simulink model "Final_Model"  (R2020a)
settings: Solver=VariableStepAuto  StartTime=0.0  StopTime=15  RelTol=1e-3
model workspace (MAT data in the model file):
  breaker_state = Simulink.Parameter
  breaker_state.Value = 0
  breaker_state.DataType = 'auto'
  breaker_state.Dimensions = [1 1]
  cap_state = Simulink.Parameter
  cap_state.Value = 1
  cap_state.DataType = 'double'
  cap_state.Dimensions = [1 1]
undefined symbols (not defined in the file or in its folder): state
libraries: ee_lib x78, nesl_utility x49, fl_lib x10, simulink x2
(part 1 of 2)
settings Model: OrderedModelArguments=off  Creator=mrinm  LastModifiedBy=HP

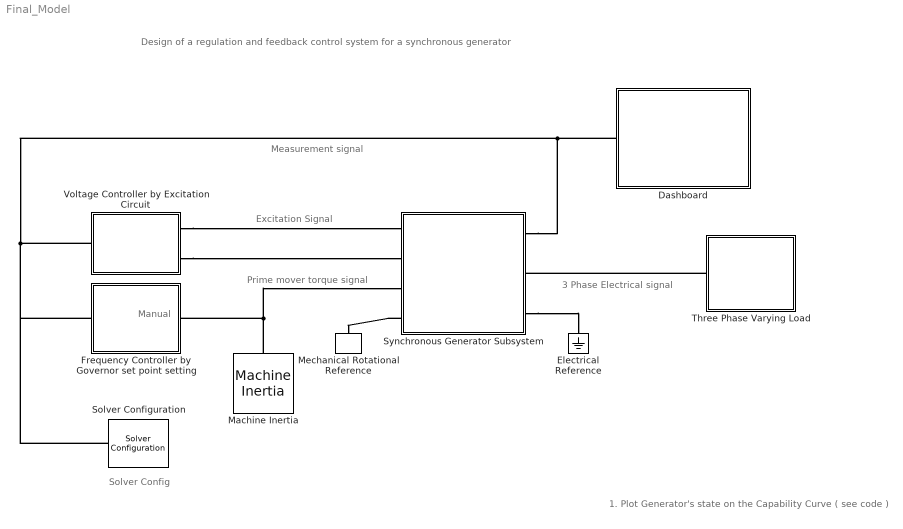
== system Final_Model ==
  note: Design of a regulation and feedback control system
      | for a synchronous generator
  note: 3 Phase Electrical signal
  note: 1. Plot Generator's state on the Capability Curve ( see code )
  note: Manual
  note: Measurement signal
  note: Excitation Signal
  note: Prime mover torque signal
  note: Solver Config
  Dashboard : Subsystem
      mask Display: image("images/dashboard.png")
  Electrical Reference : fl_lib/Electrical/Electrical Elements/Electrical Reference
      settings: SourceProductBaseCode=MT,SS
  Frequency Controller by Governor set point setting : Subsystem  mask(Governor and Prime Mover){pu_speed_reference=1, droop_percentage=10, T_G=0.2, T_CH=0.3, base_torque=2.65258e+06, pu_torque0=0.451059}
      mask prompts: pu_speed_reference "Speed reference, (pu)"; droop_percentage "Percentage droop, (%)"; T_G "Time constant of governor, (s)"; T_CH "Time constant of turbine T_CH, (s)"; base_torque "Base torque, (N*m)"; pu_torque0 "Initial torque, (pu)"
      mask help:
      | Implements a synchronous machine governor and prime mover.
      |
      | The governor response is modelled by a 1st order transfer function with time constant T_G. Likewise the prime mover also is a modelled by 1st order transfer function with time constant T_CH.
      |
      | The input to the block is a per-unit synchronous machine measurement vector.
      |
      | R and C are mechanical rotational ports.
      |
      | The stabilization of the rotor speed is implemented by a discrete PID controller which takes a reference speed and the pu_rotor_speed as input to calculate optimum governor set point value. The PID controller was tuned with Simulink auto tuner beforehand.
  Machine Inertia : ee_lib/Electromechanical/Mechanical/Machine Inertia  SRated=555e6 V*A  FRated=60 Hz  nPolePairs=1  inertia_option=2  J=27548 kg*m^2  H=3.525 s*W/V/A  damper_option=2  D=39.0509 N*m/(rad/s)  pu_D=0.01  initialization_option=2  fMechanical0=60 Hz  fElectrical0=60 Hz
      settings: SourceProductBaseCode=PS  InternalSimscapePortConfiguration="{\"Bottom\":[],\"Left\":[{\"id\":\"R\",\"label\":\"R\",\"type\":\"foundation.mechanical.rotational.rotational\"}],\"Right\":[],\"Top\":[]}"
  Mechanical Rotational Reference : fl_lib/Mechanical/Rotational Elements/Mechanical Rotational Reference
      settings: SourceProductBaseCode=MT,SS
  Solver Configuration : nesl_utility/Solver Configuration  PhysicalDomain=network_engine_domain  SubClassName=solver  LeftPortType=input  RightPortType=generic  Tones=[]  Harmonics=[]  SimulateNoise=off  Profile=off  UseLocalSampling=off  EnableSwitchedLinearOptims=on  FrequencyDomain=off  UseCCode=off  RelTol=0.001  AbsTol=1e-06  MinStep=1e-09  ToWorkspace=off  RevertToSquareIcSolve=off  NumHomotopyIterations=100  PhasorMode=off  PhasorModeNumHarmonics=1  DoDC=off  ResidualTolerance=1e-09  UseLocalSolver=on  LocalSolverChoice=NE_BACKWARD_EULER_ADVANCER  LocalSolverSampleTime=1e-3  DoFixedCost=on  MaxNonlinIter=3  MaxModeIter=2  LinearAlgebra=auto  EquationFormulation=NE_TIME_EF  DelaysMemoryBudget=1024  AutomaticFiltering=on  FilteringTimeConstant=0.001  PartitionStorageMethod=AS_NEEDED  PartitionMemoryBudget=1024  PartitionMethod=FAST
      settings: SourceProductBaseCode=MT,SS
  Synchronous Generator Subsystem : Subsystem
      mask Display: image("images/generator.jpg")
  Three Phase Varying Load : Subsystem  mask{load_type=3.Increasing Lagging, vrated=24e3, frated=60, varated=555e6}
      mask prompts: load_type "Select Load"; vrated "Rated Voltage"; frated "Rated Frequency"; varated "VA ratings"
      mask help:
      | The 3 phase load is a combination of multiple loads seen in a typical power system. A practical load is a function of time. The loads are modeled in this component.The load types are:
      | 1. Increasing Unity: A load with unity powerfactor and increasing magnitude(VA)
      | 2. Increasing Leading: A fully leading load with increasing magnitude(VA)
      | 3. Increasing Lagging: A fully lagging load with increasing magnitude(VA)
      | 4. Leading to Lagging: A load with increasing powerfactor
      | 5. Lagging to Leading: A load with decreasing powerfactor
      | 6. Varying Load: A load which VA is changing over time.
      | 7. Overload: A load bigger than the rated load.
      |
      | (Loads are not continuously time varying. Their variation is discrete.)
      mask init:
      | global state
      mask TypeOptions load_type: 1.Increasing Unity | 2.Increasing Leading | 3.Increasing Lagging | 4.Leading to Lagging | 5.Lagging to Leading | 6.Varying load | 7.Overload
      mask Callback load_type:
      | maskStr = get_param(gcb,'load_type');
      | global state
      | state=[1 1 1 1 1 1 1 1 1 1];
      | % The pop-up menu is the first mask parameter.
      | %   Check the value selected in the pop-up
      | if strcmp(maskStr(1),'1'),
      |     state(1) = 0;
      | elseif strcmp(maskStr(1),'2'),
      |     state(2) = 0;
      | elseif strcmp(maskStr(1),'3'),
      |     state(3) = 0;
      | elseif strcmp(maskStr(1),'4'),
      |     state(4) = 0;
      | elseif strcmp(maskStr(1),'5'),
      |     state(5) = 0;
      | elseif strcmp(maskStr(1),'6'),
      |     state(6) = 0;
      | elseif strcmp(maskStr(1),'7'),
      |     state(7) = 0;
      | elseif strcmp(maskStr(1),'8'),
      |     state(8) = 0;
      | elseif strcmp(maskStr(1),'9'),
      |     state(9) = 0;
      | else
      |     state(10) = 0;
      | 
      |     % Turn off the visibility of the Value field
      |     %   when User-defined is not selected.
      | 
      | 
      | 
      |     % Set the character vector in the Values field equal to the
      |     % character vector selected in the Gain pop-up menu.
      | 
      |     %maskStr{2}=maskStr{1};
      |     %set_param(gcb,'editvalue',maskStr);
      | end
      | disp(state);
      mask Display: image("images/electric_load.jpg")
  Voltage Controller by Excitation Circuit : Subsystem  mask{Vref=1, Tr=0, Ka=50, Ta=0.070, Kf=0.05, Tf=1.040, Te=0.703}
      mask prompts: Vref "Reference Voltage Vref(pu)"; Tr "Tranducer Time Constant Tr(s)"; Ka "Regulator Gain Ka(10-400)"; Ta "AVR Time Constant Ta(s)"; Kf "Feedback Gain Kf(0.03-0.1)"; Tf "Feedback Time Constant Tf(s)"; Te "Exciter Time Constant Te(s)"
      mask DialogControl DescGroupVar Prompt: Voltage Controller(mask)
      mask DialogControl DescTextVar Prompt: The input to the block is a per-unit synchronous machine measurement vector. fd+ & fd- are the positive & negative terminal field voltage
  connections:
  Machine Inertia/LConn1 -- Synchronous Generator Subsystem/LConn3 -- Frequency Controller by Governor set point setting/RConn1
  Synchronous Generator Subsystem/RConn1 -- Frequency Controller by Governor set point setting/LConn1 -- Solver Configuration/RConn1 -- Voltage Controller by Excitation Circuit/LConn1 -- Dashboard/LConn1
  Voltage Controller by Excitation Circuit/RConn1 -- Synchronous Generator Subsystem/LConn1
  Voltage Controller by Excitation Circuit/RConn2 -- Synchronous Generator Subsystem/LConn2
  Synchronous Generator Subsystem/LConn4 -- Mechanical Rotational Reference/LConn1
  Synchronous Generator Subsystem/RConn3 -- Electrical Reference/LConn1
  Three Phase Varying Load/LConn1 -- Synchronous Generator Subsystem/RConn2

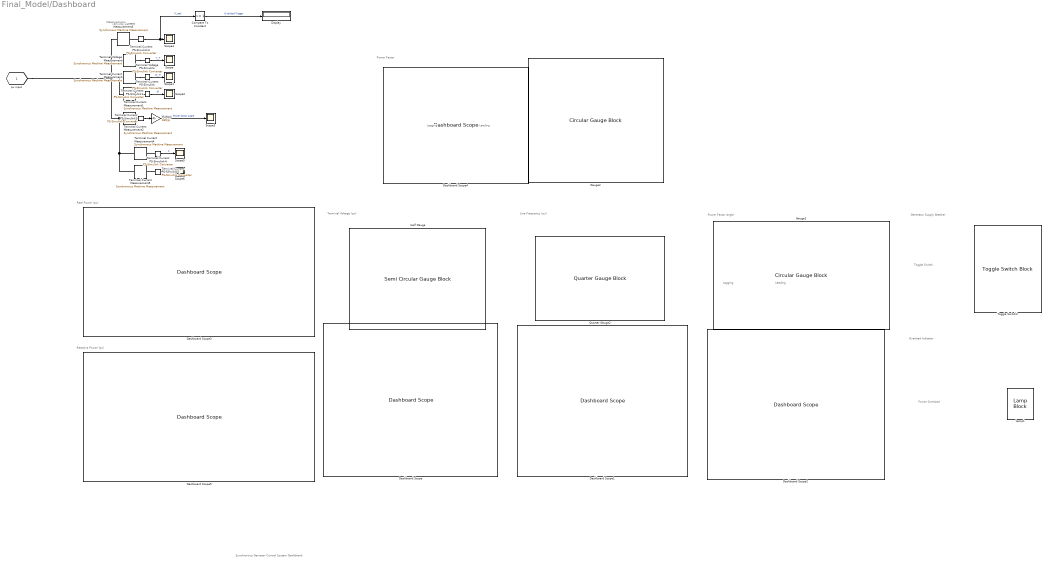
== system Final_Model/Dashboard ==
  note: Power Overload
  note: Lagging
  note: Leading
  note: Terminal Voltage (pu)
  note: Line Frequency (pu)
  note: Synchronous Genrator Control System Dashboard
  note: Power Factor Angle
  note: Leading
  note: Lagging
  note: Power Factor
  note: Real Power (pu)
  note: Overload Indicator
  note: Generator Supply Breaker
  note: Measurement
  note: Toggle Switch
  note: Reactive Power (pu)
  Compare To Constant : simulink/Logic and Bit Operations/Compare To Constant  relop=>=  const=1  OutDataTypeStr=uint8
  Dashboard Scope : DashboardScope  Ymin=0  Ymax=2  LegendPosition=Hide  ScaleAtStop=off
  Dashboard Scope1 : DashboardScope  Ymin=.9  Ymax=1.1  LegendPosition=Hide  ScaleAtStop=off
  Dashboard Scope2 : DashboardScope  Ymin=-90  Ymax=90  LegendPosition=Hide  ScaleAtStop=off
  Dashboard Scope3 : DashboardScope  Ymin=0  Ymax=2  ScaleAtStop=off
  Dashboard Scope4 : DashboardScope  Ymin=0  Ymax=1.2  LegendPosition=Hide  ScaleAtStop=off
  Dashboard Scope5 : DashboardScope  Ymin=-2  Ymax=2  ScaleAtStop=off
  Display : Display
  Gauge1 : CircularGaugeBlock  LabelPosition=Hide  ScaleMin=-90  ScaleMax=90  TickInterval=20
  Gauge2 : CircularGaugeBlock  LabelPosition=Hide  ScaleMax=1  TickInterval=0.1
  Half Gauge : SemiCircularGaugeBlock  ScaleMin=.5  ScaleMax=1.3  TickInterval=0.1
  Lamp1 : LampBlock  LabelPosition=Hide
  Multiply : Gain  Gain=180/pi
  Quarter Gauge2 : QuarterGaugeBlock  ScaleMin=.8  ScaleMax=1.2  TickInterval=.1
  Scope{,1..6} (7 alike) : Scope
  Terminal Current Measurement : ee_lib/Electromechanical/Synchronous/Synchronous Machine Measurement  output_idx=4
      settings: SourceProductBaseCode=PS  InternalSimscapePortConfiguration="{\"Bottom\":[],\"Left\":[{\"id\":\"pu_input\",\"label\":\"pu\",\"type\":\"input\"}],\"Right\":[{\"id\":\"pu_output\",\"label\":\"o\",\"type\":\"output\"}],\"Top\":[]}"
  Terminal Current Measurement1 : ee_lib/Electromechanical/Synchronous/Synchronous Machine Measurement  output_idx=17
      settings: SourceProductBaseCode=PS  InternalSimscapePortConfiguration="{\"Bottom\":[],\"Left\":[{\"id\":\"pu_input\",\"label\":\"pu\",\"type\":\"input\"}],\"Right\":[{\"id\":\"pu_output\",\"label\":\"o\",\"type\":\"output\"}],\"Top\":[]}"
  Terminal Current Measurement2 : ee_lib/Electromechanical/Synchronous/Synchronous Machine Measurement  output_idx=16
      settings: SourceProductBaseCode=PS  InternalSimscapePortConfiguration="{\"Bottom\":[],\"Left\":[{\"id\":\"pu_input\",\"label\":\"pu\",\"type\":\"input\"}],\"Right\":[{\"id\":\"pu_output\",\"label\":\"o\",\"type\":\"output\"}],\"Top\":[]}"
  Terminal Current Measurement3 : ee_lib/Electromechanical/Synchronous/Synchronous Machine Measurement  output_idx=12
      settings: SourceProductBaseCode=PS  InternalSimscapePortConfiguration="{\"Bottom\":[],\"Left\":[{\"id\":\"pu_input\",\"label\":\"pu\",\"type\":\"input\"}],\"Right\":[{\"id\":\"pu_output\",\"label\":\"o\",\"type\":\"output\"}],\"Top\":[]}"
  Terminal Current Measurement4 : ee_lib/Electromechanical/Synchronous/Synchronous Machine Measurement  output_idx=12
      settings: SourceProductBaseCode=PS  InternalSimscapePortConfiguration="{\"Bottom\":[],\"Left\":[{\"id\":\"pu_input\",\"label\":\"pu\",\"type\":\"input\"}],\"Right\":[{\"id\":\"pu_output\",\"label\":\"o\",\"type\":\"output\"}],\"Top\":[]}"
  Terminal Current Measurement5 : ee_lib/Electromechanical/Synchronous/Synchronous Machine Measurement  output_idx=13
      settings: SourceProductBaseCode=PS  InternalSimscapePortConfiguration="{\"Bottom\":[],\"Left\":[{\"id\":\"pu_input\",\"label\":\"pu\",\"type\":\"input\"}],\"Right\":[{\"id\":\"pu_output\",\"label\":\"o\",\"type\":\"output\"}],\"Top\":[]}"
  Terminal Current PS-Simulink{,1..5} (6 alike) : nesl_utility/PS-Simulink Converter  PhysicalDomain=network_engine_domain  SubClassName=ps_output  LeftPortType=input  RightPortType=output  PseudoPeriodic=off  Frequencies=[]  Unit=1  AffineConversion=off
      settings: SourceProductBaseCode=MT,SS
  Terminal Voltage Measurement : ee_lib/Electromechanical/Synchronous/Synchronous Machine Measurement  output_idx=14
      settings: SourceProductBaseCode=PS  InternalSimscapePortConfiguration="{\"Bottom\":[],\"Left\":[{\"id\":\"pu_input\",\"label\":\"pu\",\"type\":\"input\"}],\"Right\":[{\"id\":\"pu_output\",\"label\":\"o\",\"type\":\"output\"}],\"Top\":[]}"
  Terminal Voltage PS-Simulink : nesl_utility/PS-Simulink Converter  PhysicalDomain=network_engine_domain  SubClassName=ps_output  LeftPortType=input  RightPortType=output  PseudoPeriodic=off  Frequencies=[]  Unit=1  AffineConversion=off
      settings: SourceProductBaseCode=MT,SS
  Toggle Switch3 : ToggleSwitchBlock  LabelPosition=Hide
      settings: Values={{'Off', 'On'}, [1 0]}
  pu input : PMIOPort  Side=Left
  wires:
  Terminal Current PS-Simulink/1 -> Scope1/1  "W_m"
  Terminal Voltage PS-Simulink/1 -> Scope/1  "V_T"
  Compare To Constant/1 -> Display/1  "Overload Trigger"
  Terminal Current PS-Simulink1/1 -> Scope2/1  "pf"
  Terminal Current PS-Simulink3/1 -> Compare To Constant/1, Scope4/1  "P_real"
  Terminal Current PS-Simulink2/1 -> Multiply/1
  Multiply/1 -> Scope3/1  "Power factor angle"
  Terminal Current PS-Simulink4/1 -> Scope5/1  "P"
  Terminal Current PS-Simulink5/1 -> Scope6/1  "Q"
  connections:
  Terminal Current Measurement1/LConn1 -- Terminal Current Measurement/LConn1 -- Terminal Current Measurement5/LConn1 -- Terminal Current Measurement4/LConn1 -- Terminal Current Measurement2/LConn1 -- pu input/RConn1 -- Terminal Current Measurement3/LConn1 -- Terminal Voltage Measurement/LConn1
  Terminal Current PS-Simulink3/LConn1 -- Terminal Current Measurement3/RConn1
  Terminal Current PS-Simulink1/LConn1 -- Terminal Current Measurement1/RConn1
  Terminal Current PS-Simulink2/LConn1 -- Terminal Current Measurement2/RConn1
  Terminal Current Measurement/RConn1 -- Terminal Current PS-Simulink/LConn1
  Terminal Voltage Measurement/RConn1 -- Terminal Voltage PS-Simulink/LConn1
  Terminal Current PS-Simulink4/LConn1 -- Terminal Current Measurement4/RConn1
  Terminal Current PS-Simulink5/LConn1 -- Terminal Current Measurement5/RConn1

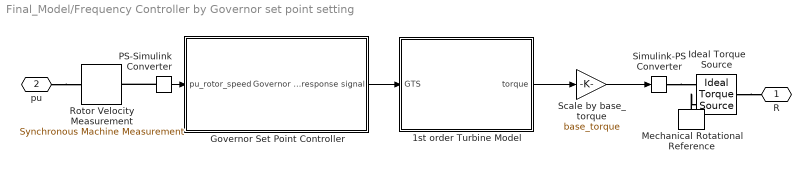
== system Final_Model/Frequency Controller by Governor set point setting ==
  1st order Turbine Model : Subsystem
  Governor Set Point Controller : Subsystem
  Ideal Torque Source : fl_lib/Mechanical/Mechanical Sources/Ideal Torque Source
      settings: SourceProductBaseCode=MT,SS
  Mechanical Rotational Reference : fl_lib/Mechanical/Rotational Elements/Mechanical Rotational Reference
      settings: SourceProductBaseCode=MT,SS
  PS-Simulink Converter : nesl_utility/PS-Simulink Converter  PhysicalDomain=network_engine_domain  SubClassName=ps_output  LeftPortType=input  RightPortType=output  PseudoPeriodic=off  Frequencies=[]  Unit=1  AffineConversion=off
      settings: SourceProductBaseCode=MT,SS
  Rotor Velocity Measurement : ee_lib/Electromechanical/Synchronous/Synchronous Machine Measurement  output_idx=4
      settings: SourceProductBaseCode=PS  InternalSimscapePortConfiguration="{\"Bottom\":[],\"Left\":[{\"id\":\"pu_input\",\"label\":\"pu\",\"type\":\"input\"}],\"Right\":[{\"id\":\"pu_output\",\"label\":\"o\",\"type\":\"output\"}],\"Top\":[]}"
  Scale by base_torque : Gain  Gain=base_torque
  Simulink-PS Converter : nesl_utility/Simulink-PS Converter  PhysicalDomain=network_engine_domain  SubClassName=ps_input  LeftPortType=input  RightPortType=output  PseudoPeriodic=off  Frequencies=[]  NoiseDistribution=none  NoiseParameters=[]  Unit=1  AffineConversion=off  FilteringAndDerivatives=zero  SimscapeFilterOrder=1  InputFilterTimeConstant=0.001  UdotUserProvided=1
      settings: SourceProductBaseCode=MT,SS
  R : PMIOPort  Side=Right
  pu : PMIOPort  Port=2  Side=Left
  wires:
  PS-Simulink Converter/1 -> Governor Set Point Controller/1(pu_rotor_speed)
  Scale by base_torque/1 -> Simulink-PS Converter/1
  1st order Turbine Model/1(torque) -> Scale by base_torque/1
  Governor Set Point Controller/1(Governor response signal) -> 1st order Turbine Model/1(GTS)
  connections:
  Mechanical Rotational Reference/LConn1 -- Ideal Torque Source/RConn2
  Ideal Torque Source/LConn1 -- R/RConn1
  pu/RConn1 -- Rotor Velocity Measurement/LConn1
  PS-Simulink Converter/LConn1 -- Rotor Velocity Measurement/RConn1
  Simulink-PS Converter/RConn1 -- Ideal Torque Source/RConn1

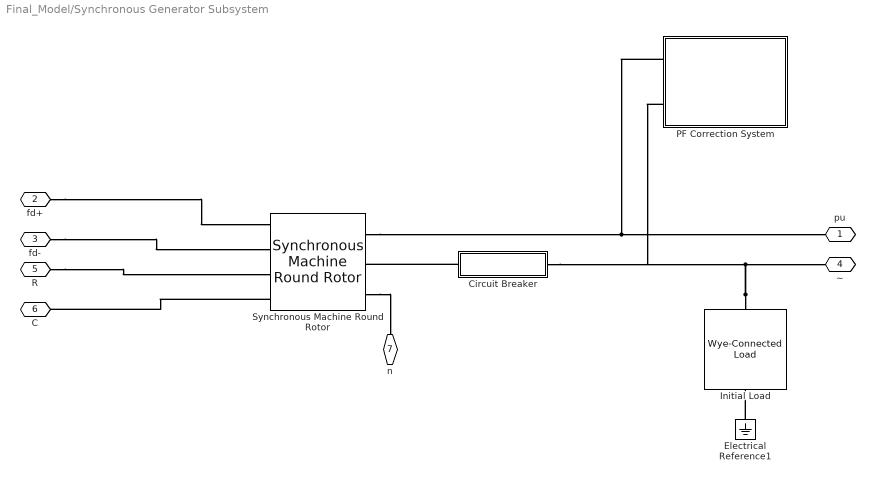
== system Final_Model/Synchronous Generator Subsystem ==
  Circuit Breaker : Subsystem
  Electrical Reference1 : fl_lib/Electrical/Electrical Elements/Electrical Reference
      settings: SourceProductBaseCode=MT,SS
  Initial Load : ee_lib/Passive/RLC Assemblies/Wye-Connected Load  parameterization=2  component_structure=1  component_structure_PQ=1  R=1 Ohm  L=0.001 H  C=1e-6 F  IL0=[ 0 0 0 ] A  VC0=[ 0 0 0 ] V  R_parasitic=1e-6 Ohm  G_parasitic=1e-6 1/Ohm  VRated=24e3 V  FRated=60 Hz  P=150e6 W  Qpos=0 V*A  Qneg=-500e6 V*A  Vmag0=2.4e+4 V  Vang0=0 deg  Freq0=60 Hz  R_parasitic_PQ=1e-6 Ohm  G_parasitic_PQ=1e-6 1/Ohm
      settings: SourceProductBaseCode=PS
  PF Correction System : Subsystem  mask{transport_delay=1, cap_reactive_power=-55e6, cut_off_pf=0.9}
      mask prompts: transport_delay "Time delay for connecting the Capacitor Bank"; cap_reactive_power "Reactive Power Delivered by the Capcitor Bank (VAR)"; cut_off_pf "Cut-off Power Factor"
      mask DialogControl DescGroupVar Prompt: PF Correction
  Synchronous Machine Round Rotor : ee_lib/Electromechanical/Synchronous/Synchronous Machine Round Rotor  SRated=555e6 V*A  VRated=24e3 V  FRated=60 Hz  nPolePairs=1  param_option=ee.enum.sm.parameterization.standard  fieldCircuitParameterization_option=ee.enum.sm.fieldparameterization.current  baseEfd=92.95 V  baseIfd=1300 A  zero_sequence=ee.enum.park.zerosequence.include  Ladu=1.66  Laqu=1.61  L0=0.15  Ll=0.15  Ra=0.003  Lfd=0.165  Rfd=0.0006  L1d=0.1713  R1d=0.0284  L1q=0.7252  R1q=0.00619  L2q=0.125  R2q=0.02368  Xl=0.15  Xd=1.81  Xq=1.76  X0=0.15  Xdd=0.3  Xqd=0.65  Xddd=0.23  Xqdd=0.25  d_option=ee.enum.circuit.open  Td0d=8 s  Tdd=1.3260 s  Td0dd=0.03 s  Tddd=0.0230 s  q_option=ee.enum.circuit.open  Tq0d=1 s  Tqd=0.3693 s  Tq0dd=0.07 s  Tqdd=0.0269 s  saturation_option=ee.enum.saturation.exclude  axes_param=ee.enum.rotorangle.daxis  saturation_ifd=[0.00, 0.48, 0.76, 1.38, 1.79]  saturation_Vag=[0.00, 0.80, 1.08, 1.31, 1.40]  initialization_option=ee.enum.sm.initialization.electrical  source_type=ee.enum.sm.load_flow_source_type.Swing  Vmag0=24e3 V  Vang0=0 deg  Pt0=150e6 V*A  Qt0=0 V*A  minimum_pu=0.95  phase_search_range=[-30, 30] deg  gmin=1e-6 S  connection_option=ee.enum.Connection.wye  num_q_dampers=2  rotor_offset=-pi / 2 rad  pu_psid_specify=on  pu_psid_priority=High  pu_psid=0  pu_psid_nominal_specify=off  pu_psid_nominal_unit=1  pu_psid_nominal_value=1  pu_psiq_specify=on  pu_psiq_priority=High  pu_psiq=0  pu_psiq_nominal_specify=off  pu_psiq_nominal_unit=1  pu_psiq_nominal_value=1  pu_psifd_specify=on  pu_psifd_priority=High  pu_psifd=0  pu_psifd_nominal_specify=off  pu_psifd_nominal_unit=1  pu_psifd_nominal_value=1  pu_psi1d_specify=on  pu_psi1d_priority=High  pu_psi1d=0  pu_psi1d_nominal_specify=off  pu_psi1d_nominal_unit=1  pu_psi1d_nominal_value=1  pu_psi1q_specify=on  pu_psi1q_priority=High  pu_psi1q=0  pu_psi1q_nominal_specify=off  pu_psi1q_nominal_unit=1  pu_psi1q_nominal_value=1  pu_psi2q_specify=on  pu_psi2q_priority=High  pu_psi2q=0  pu_psi2q_nominal_specify=off  pu_psi2q_nominal_unit=1  pu_psi2q_nominal_value=1  angular_position_diff_specify=on  angular_position_diff_priority=High  angular_position_diff=0 deg  angular_position_diff_nominal_specify=off  angular_position_diff_nominal_unit=deg  angular_position_diff_nominal_value=1
      settings: SourceProductBaseCode=PS  InternalSimscapePortConfiguration="{\"Bottom\":[],\"Left\":[{\"id\":\"fd_p\",\"label\":\"fd+\",\"type\":\"foundation.electrical.electrical\"},{\"id\":\"fd_n\",\"label\":\"fd-\",\"type\":\"foundation.electrical.electrical\"},{\"id\":\"R\",\"label\":\"R\",\"type\":\"foundation.mechanical.rotational.rotational\"},{\"id\":\"C\",\"label\":\"C\",\"type\":\"foundation.mechanical.rotational.rotational\"}],\"Right\":[{\"id\":\"pu_output\",\"label\":\"pu\",\"type\":\"output\"},{\"id\":\"N\",\"label\":\"~\",\"type\":\"foundation.electrical.three_phase\"},{\"id\":\"n\",\"label\":\"n\",\"type\":\"foundation.electrical.electrical\"}],\"Top\":[]}"
  pu : PMIOPort  Side=Right
  fd+ : PMIOPort  Port=2  Side=Left
  fd- : PMIOPort  Port=3  Side=Left
  ~ : PMIOPort  Port=4  Side=Right
  R : PMIOPort  Port=5  Side=Left
  C : PMIOPort  Port=6  Side=Left
  n : PMIOPort  Port=7  Side=Right
  connections:
  R/RConn1 -- Synchronous Machine Round Rotor/LConn3
  Synchronous Machine Round Rotor/RConn3 -- n/RConn1
  fd+/RConn1 -- Synchronous Machine Round Rotor/LConn1
  Synchronous Machine Round Rotor/LConn4 -- C/RConn1
  Synchronous Machine Round Rotor/RConn1 -- PF Correction System/LConn1 -- pu/RConn1
  fd-/RConn1 -- Synchronous Machine Round Rotor/LConn2
  Initial Load/LConn1 -- Circuit Breaker/RConn1 -- PF Correction System/LConn2 -- ~/RConn1
  Electrical Reference1/LConn1 -- Initial Load/RConn1
  Circuit Breaker/LConn1 -- Synchronous Machine Round Rotor/RConn2

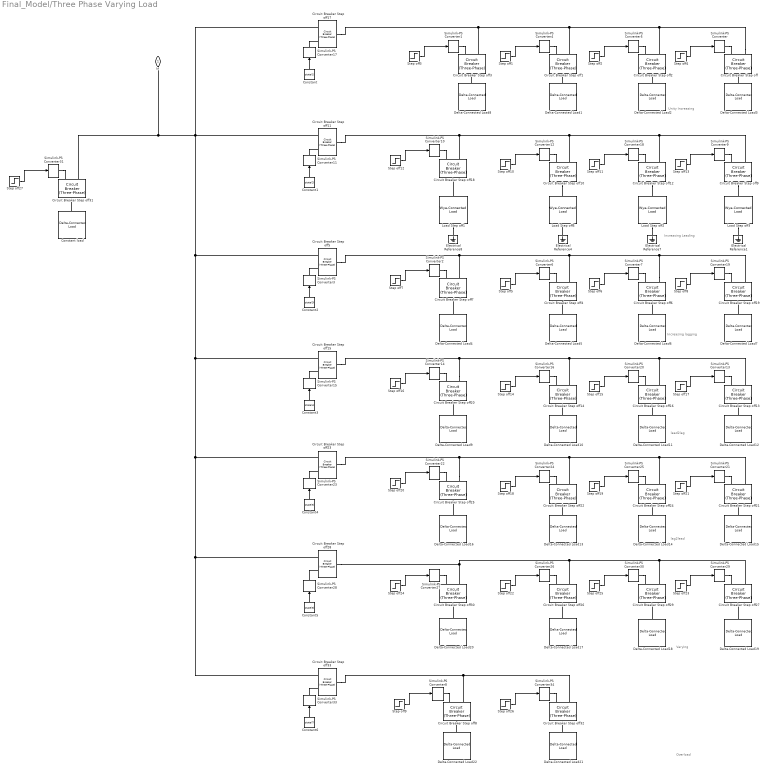
== system Final_Model/Three Phase Varying Load ==
  note: Overload
  note: Unity Increasing
  note: Increasing Leading
  note: Increasing lagging
  note: lead2lag
  note: lag2lead
  note: Varying
  Circuit Breaker Step off{,1..33} (34 alike) : ee_lib/Switches & Breakers/Circuit Breaker (Three-Phase)  R_closed=0.001 Ohm  G_open=1e-4 1/Ohm  threshold=0.5 V
      settings: SourceProductBaseCode=PS  InternalSimscapePortConfiguration="{\"Bottom\":[],\"Left\":[{\"id\":\"vT\",\"label\":\"vT\",\"type\":\"input\"},{\"id\":\"N1\",\"label\":\"~1\",\"type\":\"foundation.electrical.three_phase\"}],\"Right\":[{\"id\":\"N2\",\"label\":\"~2\",\"type\":\"foundation.electrical.three_phase\"}],\"Top\":[]}"
  Constant : Constant  Value=state(1)
  Constant load : ee_lib/Passive/RLC Assemblies/Delta-Connected Load  parameterization=2  component_structure=1  component_structure_PQ=11  R=1 Ohm  L=0.001 H  C=1e-6 F  IL0=[ 0 0 0 ] A  VC0=[ 0 0 0 ] V  R_parasitic=1e-6 Ohm  G_parasitic=1e-6 1/Ohm  VRated=vrated V  FRated=frated Hz  P=0.4*varated W  Qpos=0.001*varated V*A  Qneg=-0.001*varated V*A  Vmag0=2.4e+4 V  Vang0=0 deg  Freq0=60 Hz  R_parasitic_PQ=1e-6 Ohm  G_parasitic_PQ=1e-6 1/Ohm
      settings: SourceProductBaseCode=PS  InternalSimscapePortConfiguration="{\"Bottom\":[],\"Left\":[{\"id\":\"N\",\"label\":\"~\",\"type\":\"foundation.electrical.three_phase\"}],\"Right\":[],\"Top\":[]}"
  Constant1 : Constant  Value=state(2)
  Constant2 : Constant  Value=state(3)
  Constant3 : Constant  Value=state(4)
  Constant4 : Constant  Value=state(5)
  Constant5 : Constant  Value=state(6)
  Constant6 : Constant  Value=state(7)
  Delta-Connected Load1 : ee_lib/Passive/RLC Assemblies/Delta-Connected Load  parameterization=2  component_structure=1  component_structure_PQ=1  R=1 Ohm  L=0.001 H  C=1e-6 F  IL0=[ 0 0 0 ] A  VC0=[ 0 0 0 ] V  R_parasitic=1e-6 Ohm  G_parasitic=1e-6 1/Ohm  VRated=vrated V  FRated=60 Hz  P=0.1*varated W  Qpos=100 V*A  Qneg=-100 V*A  Vmag0=2.4e+4 V  Vang0=0 deg  Freq0=60 Hz  R_parasitic_PQ=1e-6 Ohm  G_parasitic_PQ=1e-6 1/Ohm
      settings: SourceProductBaseCode=PS  InternalSimscapePortConfiguration="{\"Bottom\":[],\"Left\":[{\"id\":\"N\",\"label\":\"~\",\"type\":\"foundation.electrical.three_phase\"}],\"Right\":[],\"Top\":[]}"
  Delta-Connected Load{4,10..12} (4 alike) : ee_lib/Passive/RLC Assemblies/Delta-Connected Load  parameterization=2  component_structure=1  component_structure_PQ=4  R=1 Ohm  L=0.001 H  C=1e-6 F  IL0=[ 0 0 0 ] A  VC0=[ 0 0 0 ] V  R_parasitic=1e-6 Ohm  G_parasitic=1e-6 1/Ohm  VRated=vrated V  FRated=frated Hz  P=10 W  Qpos=0.1*varated V*A  Qneg=-100 V*A  Vmag0=2.4e+4 V  Vang0=0 deg  Freq0=60 Hz  R_parasitic_PQ=1e-6 Ohm  G_parasitic_PQ=1e-6 1/Ohm
      settings: SourceProductBaseCode=PS  InternalSimscapePortConfiguration="{\"Bottom\":[],\"Left\":[{\"id\":\"N\",\"label\":\"~\",\"type\":\"foundation.electrical.three_phase\"}],\"Right\":[],\"Top\":[]}"
  Delta-Connected Load13 : ee_lib/Passive/RLC Assemblies/Delta-Connected Load  parameterization=2  component_structure=1  component_structure_PQ=5  R=1 Ohm  L=0.001 H  C=1e-6 F  IL0=[ 0 0 0 ] A  VC0=[ 0 0 0 ] V  R_parasitic=1e-6 Ohm  G_parasitic=1e-6 1/Ohm  VRated=vrated V  FRated=frated Hz  P=10 W  Qpos=10e6 V*A  Qneg=-0.1*varated V*A  Vmag0=2.4e+4 V  Vang0=0 deg  Freq0=60 Hz  R_parasitic_PQ=1e-6 Ohm  G_parasitic_PQ=1e-6 1/Ohm
      settings: SourceProductBaseCode=PS  InternalSimscapePortConfiguration="{\"Bottom\":[],\"Left\":[{\"id\":\"N\",\"label\":\"~\",\"type\":\"foundation.electrical.three_phase\"}],\"Right\":[],\"Top\":[]}"
  Delta-Connected Load14 : ee_lib/Passive/RLC Assemblies/Delta-Connected Load  parameterization=2  component_structure=1  component_structure_PQ=5  R=1 Ohm  L=0.001 H  C=1e-6 F  IL0=[ 0 0 0 ] A  VC0=[ 0 0 0 ] V  R_parasitic=1e-6 Ohm  G_parasitic=1e-6 1/Ohm  VRated=vrated V  FRated=frated Hz  P=10 W  Qpos=10e6 V*A  Qneg=-0.1*varated V*A  Vmag0=2.4e+4 V  Vang0=0 deg  Freq0=60 Hz  R_parasitic_PQ=1e-6 Ohm  G_parasitic_PQ=1e-6 1/Ohm
      settings: SourceProductBaseCode=PS  InternalSimscapePortConfiguration="{\"Bottom\":[],\"Left\":[{\"id\":\"N\",\"label\":\"~\",\"type\":\"foundation.electrical.three_phase\"}],\"Right\":[],\"Top\":[]}"
  Delta-Connected Load15 : ee_lib/Passive/RLC Assemblies/Delta-Connected Load  parameterization=2  component_structure=1  component_structure_PQ=5  R=1 Ohm  L=0.001 H  C=1e-6 F  IL0=[ 0 0 0 ] A  VC0=[ 0 0 0 ] V  R_parasitic=1e-6 Ohm  G_parasitic=1e-6 1/Ohm  VRated=vrated V  FRated=frated Hz  P=10 W  Qpos=10e6 V*A  Qneg=-0.1*varated V*A  Vmag0=2.4e+4 V  Vang0=0 deg  Freq0=60 Hz  R_parasitic_PQ=1e-6 Ohm  G_parasitic_PQ=1e-6 1/Ohm
      settings: SourceProductBaseCode=PS  InternalSimscapePortConfiguration="{\"Bottom\":[],\"Left\":[{\"id\":\"N\",\"label\":\"~\",\"type\":\"foundation.electrical.three_phase\"}],\"Right\":[],\"Top\":[]}"
  Delta-Connected Load16 : ee_lib/Passive/RLC Assemblies/Delta-Connected Load  parameterization=2  component_structure=1  component_structure_PQ=8  R=1 Ohm  L=0.001 H  C=1e-6 F  IL0=[ 0 0 0 ] A  VC0=[ 0 0 0 ] V  R_parasitic=1e-6 Ohm  G_parasitic=1e-6 1/Ohm  VRated=vrated V  FRated=frated Hz  P=10 W  Qpos=0.1*varated V*A  Qneg=-15e6 V*A  Vmag0=2.4e+4 V  Vang0=0 deg  Freq0=60 Hz  R_parasitic_PQ=1e-6 Ohm  G_parasitic_PQ=1e-6 1/Ohm
      settings: SourceProductBaseCode=PS  InternalSimscapePortConfiguration="{\"Bottom\":[],\"Left\":[{\"id\":\"N\",\"label\":\"~\",\"type\":\"foundation.electrical.three_phase\"}],\"Right\":[],\"Top\":[]}"
  Delta-Connected Load17 : ee_lib/Passive/RLC Assemblies/Delta-Connected Load  parameterization=2  component_structure=1  component_structure_PQ=4  R=1 Ohm  L=0.001 H  C=1e-6 F  IL0=[ 0 0 0 ] A  VC0=[ 0 0 0 ] V  R_parasitic=1e-6 Ohm  G_parasitic=1e-6 1/Ohm  VRated=vrated V  FRated=frated Hz  P=0.05*varated W  Qpos=0.1*varated V*A  Qneg=-15e6 V*A  Vmag0=2.4e+4 V  Vang0=0 deg  Freq0=60 Hz  R_parasitic_PQ=1e-6 Ohm  G_parasitic_PQ=1e-6 1/Ohm
      settings: SourceProductBaseCode=PS  InternalSimscapePortConfiguration="{\"Bottom\":[],\"Left\":[{\"id\":\"N\",\"label\":\"~\",\"type\":\"foundation.electrical.three_phase\"}],\"Right\":[],\"Top\":[]}"
  Delta-Connected Load18 : ee_lib/Passive/RLC Assemblies/Delta-Connected Load  parameterization=2  component_structure=1  component_structure_PQ=4  R=1 Ohm  L=0.001 H  C=1e-6 F  IL0=[ 0 0 0 ] A  VC0=[ 0 0 0 ] V  R_parasitic=1e-6 Ohm  G_parasitic=1e-6 1/Ohm  VRated=vrated V  FRated=frated Hz  P=0.05*varated W  Qpos=0.1*varated V*A  Qneg=-15e6 V*A  Vmag0=2.4e+4 V  Vang0=0 deg  Freq0=60 Hz  R_parasitic_PQ=1e-6 Ohm  G_parasitic_PQ=1e-6 1/Ohm
      settings: SourceProductBaseCode=PS  InternalSimscapePortConfiguration="{\"Bottom\":[],\"Left\":[{\"id\":\"N\",\"label\":\"~\",\"type\":\"foundation.electrical.three_phase\"}],\"Right\":[],\"Top\":[]}"
  Delta-Connected Load19 : ee_lib/Passive/RLC Assemblies/Delta-Connected Load  parameterization=2  component_structure=1  component_structure_PQ=5  R=1 Ohm  L=0.001 H  C=1e-6 F  IL0=[ 0 0 0 ] A  VC0=[ 0 0 0 ] V  R_parasitic=1e-6 Ohm  G_parasitic=1e-6 1/Ohm  VRated=vrated V  FRated=frated Hz  P=0.05*varated W  Qpos=10e4 V*A  Qneg=-0.08*varated V*A  Vmag0=2.4e+4 V  Vang0=0 deg  Freq0=60 Hz  R_parasitic_PQ=1e-6 Ohm  G_parasitic_PQ=1e-6 1/Ohm
      settings: SourceProductBaseCode=PS  InternalSimscapePortConfiguration="{\"Bottom\":[],\"Left\":[{\"id\":\"N\",\"label\":\"~\",\"type\":\"foundation.electrical.three_phase\"}],\"Right\":[],\"Top\":[]}"
  Delta-Connected Load2 : ee_lib/Passive/RLC Assemblies/Delta-Connected Load  parameterization=2  component_structure=1  component_structure_PQ=1  R=1 Ohm  L=0.001 H  C=1e-6 F  IL0=[ 0 0 0 ] A  VC0=[ 0 0 0 ] V  R_parasitic=1e-6 Ohm  G_parasitic=1e-6 1/Ohm  VRated=vrated V  FRated=60 Hz  P=0.1*varated W  Qpos=100 V*A  Qneg=-100 V*A  Vmag0=2.4e+4 V  Vang0=0 deg  Freq0=60 Hz  R_parasitic_PQ=1e-6 Ohm  G_parasitic_PQ=1e-6 1/Ohm
      settings: SourceProductBaseCode=PS  InternalSimscapePortConfiguration="{\"Bottom\":[],\"Left\":[{\"id\":\"N\",\"label\":\"~\",\"type\":\"foundation.electrical.three_phase\"}],\"Right\":[],\"Top\":[]}"
  Delta-Connected Load20 : ee_lib/Passive/RLC Assemblies/Delta-Connected Load  parameterization=2  component_structure=1  component_structure_PQ=5  R=1 Ohm  L=0.001 H  C=1e-6 F  IL0=[ 0 0 0 ] A  VC0=[ 0 0 0 ] V  R_parasitic=1e-6 Ohm  G_parasitic=1e-6 1/Ohm  VRated=vrated V  FRated=frated Hz  P=0.005*varated W  Qpos=10e4 V*A  Qneg=-0.05*varated V*A  Vmag0=2.4e+4 V  Vang0=0 deg  Freq0=60 Hz  R_parasitic_PQ=1e-6 Ohm  G_parasitic_PQ=1e-6 1/Ohm
      settings: SourceProductBaseCode=PS  InternalSimscapePortConfiguration="{\"Bottom\":[],\"Left\":[{\"id\":\"N\",\"label\":\"~\",\"type\":\"foundation.electrical.three_phase\"}],\"Right\":[],\"Top\":[]}"
  Delta-Connected Load21 : ee_lib/Passive/RLC Assemblies/Delta-Connected Load  parameterization=2  component_structure=1  component_structure_PQ=4  R=1 Ohm  L=0.001 H  C=1e-6 F  IL0=[ 0 0 0 ] A  VC0=[ 0 0 0 ] V  R_parasitic=1e-6 Ohm  G_parasitic=1e-6 1/Ohm  VRated=vrated V  FRated=frated Hz  P=0.4*varated W  Qpos=0.1*varated V*A  Qneg=-100 V*A  Vmag0=2.4e+4 V  Vang0=0 deg  Freq0=60 Hz  R_parasitic_PQ=1e-6 Ohm  G_parasitic_PQ=1e-6 1/Ohm
      settings: SourceProductBaseCode=PS  InternalSimscapePortConfiguration="{\"Bottom\":[],\"Left\":[{\"id\":\"N\",\"label\":\"~\",\"type\":\"foundation.electrical.three_phase\"}],\"Right\":[],\"Top\":[]}"
  Delta-Connected Load22 : ee_lib/Passive/RLC Assemblies/Delta-Connected Load  parameterization=2  component_structure=1  component_structure_PQ=4  R=1 Ohm  L=0.001 H  C=1e-6 F  IL0=[ 0 0 0 ] A  VC0=[ 0 0 0 ] V  R_parasitic=1e-6 Ohm  G_parasitic=1e-6 1/Ohm  VRated=vrated V  FRated=frated Hz  P=0.2*varated W  Qpos=0.1*varated V*A  Qneg=-100 V*A  Vmag0=2.4e+4 V  Vang0=0 deg  Freq0=60 Hz  R_parasitic_PQ=1e-6 Ohm  G_parasitic_PQ=1e-6 1/Ohm
      settings: SourceProductBaseCode=PS  InternalSimscapePortConfiguration="{\"Bottom\":[],\"Left\":[{\"id\":\"N\",\"label\":\"~\",\"type\":\"foundation.electrical.three_phase\"}],\"Right\":[],\"Top\":[]}"
  Delta-Connected Load3 : ee_lib/Passive/RLC Assemblies/Delta-Connected Load  parameterization=2  component_structure=1  component_structure_PQ=1  R=1 Ohm  L=0.001 H  C=1e-6 F  IL0=[ 0 0 0 ] A  VC0=[ 0 0 0 ] V  R_parasitic=1e-6 Ohm  G_parasitic=1e-6 1/Ohm  VRated=vrated V  FRated=60 Hz  P=0.05*varated W  Qpos=100 V*A  Qneg=-100 V*A  Vmag0=2.4e+4 V  Vang0=0 deg  Freq0=60 Hz  R_parasitic_PQ=1e-6 Ohm  G_parasitic_PQ=1e-6 1/Ohm
      settings: SourceProductBaseCode=PS  InternalSimscapePortConfiguration="{\"Bottom\":[],\"Left\":[{\"id\":\"N\",\"label\":\"~\",\"type\":\"foundation.electrical.three_phase\"}],\"Right\":[],\"Top\":[]}"
  Delta-Connected Load5 : ee_lib/Passive/RLC Assemblies/Delta-Connected Load  parameterization=2  component_structure=1  component_structure_PQ=4  R=1 Ohm  L=0.001 H  C=1e-6 F  IL0=[ 0 0 0 ] A  VC0=[ 0 0 0 ] V  R_parasitic=1e-6 Ohm  G_parasitic=1e-6 1/Ohm  VRated=vrated V  FRated=frated Hz  P=varated*10e-4 W  Qpos=0.1*varated V*A  Qneg=-100 V*A  Vmag0=2.4e+4 V  Vang0=0 deg  Freq0=60 Hz  R_parasitic_PQ=1e-6 Ohm  G_parasitic_PQ=1e-6 1/Ohm
      settings: SourceProductBaseCode=PS  InternalSimscapePortConfiguration="{\"Bottom\":[],\"Left\":[{\"id\":\"N\",\"label\":\"~\",\"type\":\"foundation.electrical.three_phase\"}],\"Right\":[],\"Top\":[]}"
  Delta-Connected Load6 : ee_lib/Passive/RLC Assemblies/Delta-Connected Load  parameterization=2  component_structure=1  component_structure_PQ=4  R=1 Ohm  L=0.001 H  C=1e-6 F  IL0=[ 0 0 0 ] A  VC0=[ 0 0 0 ] V  R_parasitic=1e-6 Ohm  G_parasitic=1e-6 1/Ohm  VRated=vrated V  FRated=frated Hz  P=varated*10e-4 W  Qpos=0.1*varated V*A  Qneg=-100 V*A  Vmag0=2.4e+4 V  Vang0=0 deg  Freq0=60 Hz  R_parasitic_PQ=1e-6 Ohm  G_parasitic_PQ=1e-6 1/Ohm
      settings: SourceProductBaseCode=PS  InternalSimscapePortConfiguration="{\"Bottom\":[],\"Left\":[{\"id\":\"N\",\"label\":\"~\",\"type\":\"foundation.electrical.three_phase\"}],\"Right\":[],\"Top\":[]}"
  Delta-Connected Load7 : ee_lib/Passive/RLC Assemblies/Delta-Connected Load  parameterization=2  component_structure=1  component_structure_PQ=4  R=1 Ohm  L=0.001 H  C=1e-6 F  IL0=[ 0 0 0 ] A  VC0=[ 0 0 0 ] V  R_parasitic=1e-6 Ohm  G_parasitic=1e-6 1/Ohm  VRated=vrated V  FRated=frated Hz  P=varated*10e-4 W  Qpos=0.1*varated V*A  Qneg=-100 V*A  Vmag0=2.4e+4 V  Vang0=0 deg  Freq0=60 Hz  R_parasitic_PQ=1e-6 Ohm  G_parasitic_PQ=1e-6 1/Ohm
      settings: SourceProductBaseCode=PS  InternalSimscapePortConfiguration="{\"Bottom\":[],\"Left\":[{\"id\":\"N\",\"label\":\"~\",\"type\":\"foundation.electrical.three_phase\"}],\"Right\":[],\"Top\":[]}"
  Delta-Connected Load8 : ee_lib/Passive/RLC Assemblies/Delta-Connected Load  parameterization=2  component_structure=1  component_structure_PQ=1  R=1 Ohm  L=0.001 H  C=1e-6 F  IL0=[ 0 0 0 ] A  VC0=[ 0 0 0 ] V  R_parasitic=1e-6 Ohm  G_parasitic=1e-6 1/Ohm  VRated=vrated V  FRated=60 Hz  P=0.05*varated W  Qpos=100 V*A  Qneg=-100 V*A  Vmag0=2.4e+4 V  Vang0=0 deg  Freq0=60 Hz  R_parasitic_PQ=1e-6 Ohm  G_parasitic_PQ=1e-6 1/Ohm
      settings: SourceProductBaseCode=PS  InternalSimscapePortConfiguration="{\"Bottom\":[],\"Left\":[{\"id\":\"N\",\"label\":\"~\",\"type\":\"foundation.electrical.three_phase\"}],\"Right\":[],\"Top\":[]}"
  Delta-Connected Load9 : ee_lib/Passive/RLC Assemblies/Delta-Connected Load  parameterization=2  component_structure=1  component_structure_PQ=5  R=1 Ohm  L=0.001 H  C=1e-6 F  IL0=[ 0 0 0 ] A  VC0=[ 0 0 0 ] V  R_parasitic=1e-6 Ohm  G_parasitic=1e-6 1/Ohm  VRated=vrated V  FRated=frated Hz  P=10 W  Qpos=10e4 V*A  Qneg=-0.2*varated V*A  Vmag0=2.4e+4 V  Vang0=0 deg  Freq0=60 Hz  R_parasitic_PQ=1e-6 Ohm  G_parasitic_PQ=1e-6 1/Ohm
      settings: SourceProductBaseCode=PS  InternalSimscapePortConfiguration="{\"Bottom\":[],\"Left\":[{\"id\":\"N\",\"label\":\"~\",\"type\":\"foundation.electrical.three_phase\"}],\"Right\":[],\"Top\":[]}"
  Electrical Reference{1,4,7..8} (4 alike) : fl_lib/Electrical/Electrical Elements/Electrical Reference
  Load Step off1 : ee_lib/Passive/RLC Assemblies/Wye-Connected Load  parameterization=2  component_structure=1  component_structure_PQ=5  R=1 Ohm  L=0.001 H  C=1e-6 F  IL0=[ 0 0 0 ] A  VC0=[ 0 0 0 ] V  R_parasitic=1e-6 Ohm  G_parasitic=1e-6 1/Ohm  VRated=vrated V  FRated=frated Hz  P=10 W  Qpos=10 V*A  Qneg=-0.1*varated V*A  Vmag0=2.4e+4 V  Vang0=0 deg  Freq0=60 Hz  R_parasitic_PQ=1e-6 Ohm  G_parasitic_PQ=1e-6 1/Ohm
      settings: SourceProductBaseCode=PS
  Load Step off2 : ee_lib/Passive/RLC Assemblies/Wye-Connected Load  parameterization=2  component_structure=1  component_structure_PQ=3  R=1 Ohm  L=0.001 H  C=1e-6 F  IL0=[ 0 0 0 ] A  VC0=[ 0 0 0 ] V  R_parasitic=1e-6 Ohm  G_parasitic=1e-6 1/Ohm  VRated=vrated V  FRated=frated Hz  P=10 W  Qpos=10 V*A  Qneg=-0.1*varated V*A  Vmag0=2.4e+4 V  Vang0=0 deg  Freq0=60 Hz  R_parasitic_PQ=1e-6 Ohm  G_parasitic_PQ=1e-6 1/Ohm
      settings: SourceProductBaseCode=PS
  Load Step off3 : ee_lib/Passive/RLC Assemblies/Wye-Connected Load  parameterization=2  component_structure=1  component_structure_PQ=3  R=1 Ohm  L=0.001 H  C=1e-6 F  IL0=[ 0 0 0 ] A  VC0=[ 0 0 0 ] V  R_parasitic=1e-6 Ohm  G_parasitic=1e-6 1/Ohm  VRated=vrated V  FRated=frated Hz  P=10 W  Qpos=10 V*A  Qneg=-0.1*varated V*A  Vmag0=2.4e+4 V  Vang0=0 deg  Freq0=60 Hz  R_parasitic_PQ=1e-6 Ohm  G_parasitic_PQ=1e-6 1/Ohm
      settings: SourceProductBaseCode=PS
  Load Step off5 : ee_lib/Passive/RLC Assemblies/Wye-Connected Load  parameterization=2  component_structure=1  component_structure_PQ=3  R=1 Ohm  L=0.001 H  C=1e-6 F  IL0=[ 0 0 0 ] A  VC0=[ 0 0 0 ] V  R_parasitic=1e-6 Ohm  G_parasitic=1e-6 1/Ohm  VRated=vrated V  FRated=frated Hz  P=10 W  Qpos=10 V*A  Qneg=-0.1*varated V*A  Vmag0=2.4e+4 V  Vang0=0 deg  Freq0=60 Hz  R_parasitic_PQ=1e-6 Ohm  G_parasitic_PQ=1e-6 1/Ohm
      settings: SourceProductBaseCode=PS
  Simulink-PS Converter{,1..31,33..34} (34 alike) : nesl_utility/Simulink-PS Converter  PhysicalDomain=network_engine_domain  SubClassName=ps_input  LeftPortType=input  RightPortType=output  PseudoPeriodic=off  Frequencies=[]  NoiseDistribution=none  NoiseParameters=[]  Unit=1  AffineConversion=off  FilteringAndDerivatives=zero  SimscapeFilterOrder=1  InputFilterTimeConstant=0.001  UdotUserProvided=1
  Step off{1,5,10,14,18,25..26} (7 alike) : Step  Time=15  Before=1  After=0  SampleTime=0
  Step off{4,8,11,17,21} (5 alike) : Step  Time=25  Before=1  After=0  SampleTime=0
  Step off{3,7,12,16,20} (5 alike) : Step  Time=10  Before=1  After=0  SampleTime=0
  Step off13 : Step  Time=35  Before=1  After=0  SampleTime=0
  Step off{2,6,15,19} (4 alike) : Step  Time=20  Before=1  After=0  SampleTime=0
  Step off22 : Step  Time=20  SampleTime=0
  Step off23 : Step  Time=25  SampleTime=0
  Step off24 : Step  Time=7  Before=1  After=0  SampleTime=0
  Step off27 : Step  Time=5  Before=1  After=0  SampleTime=0
  Step off9 : Step  Time=5  Before=1  After=0  SampleTime=0
  In : PMIOPort  Side=Left
  wires:
  Step off1/1 -> Simulink-PS Converter4/1
  Step off2/1 -> Simulink-PS Converter5/1
  Step off4/1 -> Simulink-PS Converter/1
  Constant/1 -> Simulink-PS Converter17/1
  Step off13/1 -> Simulink-PS Converter9/1
  Step off12/1 -> Simulink-PS Converter10/1
  Step off10/1 -> Simulink-PS Converter12/1
  Step off11/1 -> Simulink-PS Converter18/1
  Constant1/1 -> Simulink-PS Converter11/1
  Step off7/1 -> Simulink-PS Converter2/1
  Step off8/1 -> Simulink-PS Converter19/1
  Constant2/1 -> Simulink-PS Converter3/1
  Step off6/1 -> Simulink-PS Converter7/1
  Step off5/1 -> Simulink-PS Converter6/1
  Step off15/1 -> Simulink-PS Converter20/1
  Step off17/1 -> Simulink-PS Converter13/1
  Constant3/1 -> Simulink-PS Converter15/1
  Step off14/1 -> Simulink-PS Converter16/1
  Step off16/1 -> Simulink-PS Converter14/1
  Constant4/1 -> Simulink-PS Converter23/1
  Step off20/1 -> Simulink-PS Converter22/1
  Step off18/1 -> Simulink-PS Converter24/1
  Step off21/1 -> Simulink-PS Converter21/1
  Step off19/1 -> Simulink-PS Converter25/1
  Constant5/1 -> Simulink-PS Converter28/1
  Step off24/1 -> Simulink-PS Converter27/1
  Constant6/1 -> Simulink-PS Converter33/1
  Step off26/1 -> Simulink-PS Converter34/1
  Step off22/1 -> Simulink-PS Converter26/1
  Step off23/1 -> Simulink-PS Converter29/1
  Step off25/1 -> Simulink-PS Converter30/1
  Step off3/1 -> Simulink-PS Converter1/1
  Step off9/1 -> Simulink-PS Converter8/1
  Step off27/1 -> Simulink-PS Converter31/1
  connections:
  Simulink-PS Converter4/RConn1 -- Circuit Breaker Step off1/LConn1
  Delta-Connected Load1/LConn1 -- Circuit Breaker Step off1/RConn1
  Simulink-PS Converter5/RConn1 -- Circuit Breaker Step off2/LConn1
  Delta-Connected Load2/LConn1 -- Circuit Breaker Step off2/RConn1
  Simulink-PS Converter/RConn1 -- Circuit Breaker Step off/LConn1
  Delta-Connected Load3/LConn1 -- Circuit Breaker Step off/RConn1
  Load Step off3/RConn1 -- Electrical Reference1/LConn1
  Circuit Breaker Step off9/RConn1 -- Load Step off3/LConn1
  Circuit Breaker Step off10/RConn1 -- Load Step off5/LConn1
  Circuit Breaker Step off12/RConn1 -- Load Step off2/LConn1
  Electrical Reference4/LConn1 -- Load Step off5/RConn1
  Load Step off1/RConn1 -- Electrical Reference8/LConn1
  Load Step off2/RConn1 -- Electrical Reference7/LConn1
  Circuit Breaker Step off17/LConn2 -- Circuit Breaker Step off33/LConn2 -- Circuit Breaker Step off28/LConn2 -- Circuit Breaker Step off23/LConn2 -- Circuit Breaker Step off15/LConn2 -- Circuit Breaker Step off5/LConn2 -- Circuit Breaker Step off11/LConn2 -- Circuit Breaker Step off31/LConn2 -- In/RConn1
  Circuit Breaker Step off/LConn2 -- Circuit Breaker Step off2/LConn2 -- Circuit Breaker Step off3/LConn2 -- Circuit Breaker Step off17/RConn1 -- Circuit Breaker Step off1/LConn2
  Simulink-PS Converter17/RConn1 -- Circuit Breaker Step off17/LConn1
  Circuit Breaker Step off11/RConn1 -- Circuit Breaker Step off18/LConn2 -- Circuit Breaker Step off10/LConn2 -- Circuit Breaker Step off9/LConn2 -- Circuit Breaker Step off12/LConn2
  Load Step off1/LConn1 -- Circuit Breaker Step off18/RConn1
  Simulink-PS Converter11/RConn1 -- Circuit Breaker Step off11/LConn1
  Simulink-PS Converter18/RConn1 -- Circuit Breaker Step off12/LConn1
  Simulink-PS Converter10/RConn1 -- Circuit Breaker Step off18/LConn1
  Simulink-PS Converter9/RConn1 -- Circuit Breaker Step off9/LConn1
  Simulink-PS Converter12/RConn1 -- Circuit Breaker Step off10/LConn1
  Circuit Breaker Step off6/LConn2 -- Circuit Breaker Step off5/RConn1 -- Circuit Breaker Step off7/LConn2 -- Circuit Breaker Step off4/LConn2 -- Circuit Breaker Step off19/LConn2
  Delta-Connected Load7/LConn1 -- Circuit Breaker Step off19/RConn1
  Simulink-PS Converter6/RConn1 -- Circuit Breaker Step off4/LConn1
  Simulink-PS Converter7/RConn1 -- Circuit Breaker Step off6/LConn1
  Simulink-PS Converter19/RConn1 -- Circuit Breaker Step off19/LConn1
  Delta-Connected Load5/LConn1 -- Circuit Breaker Step off4/RConn1
  Simulink-PS Converter3/RConn1 -- Circuit Breaker Step off5/LConn1
  Delta-Connected Load6/LConn1 -- Circuit Breaker Step off6/RConn1
  Simulink-PS Converter2/RConn1 -- Circuit Breaker Step off7/LConn1
  Delta-Connected Load4/LConn1 -- Circuit Breaker Step off7/RConn1
  Circuit Breaker Step off20/LConn2 -- Circuit Breaker Step off14/LConn2 -- Circuit Breaker Step off13/LConn2 -- Circuit Breaker Step off16/LConn2 -- Circuit Breaker Step off15/RConn1
  Simulink-PS Converter13/RConn1 -- Circuit Breaker Step off13/LConn1
  Simulink-PS Converter15/RConn1 -- Circuit Breaker Step off15/LConn1
  Simulink-PS Converter16/RConn1 -- Circuit Breaker Step off14/LConn1
  Delta-Connected Load10/LConn1 -- Circuit Breaker Step off14/RConn1
  Simulink-PS Converter14/RConn1 -- Circuit Breaker Step off20/LConn1
  Simulink-PS Converter20/RConn1 -- Circuit Breaker Step off16/LConn1
  Delta-Connected Load11/LConn1 -- Circuit Breaker Step off16/RConn1
  Delta-Connected Load9/LConn1 -- Circuit Breaker Step off20/RConn1
  Delta-Connected Load12/LConn1 -- Circuit Breaker Step off13/RConn1
  Circuit Breaker Step off25/LConn2 -- Circuit Breaker Step off22/LConn2 -- Circuit Breaker Step off21/LConn2 -- Circuit Breaker Step off24/LConn2 -- Circuit Breaker Step off23/RConn1
  Simulink-PS Converter22/RConn1 -- Circuit Breaker Step off25/LConn1
  Simulink-PS Converter21/RConn1 -- Circuit Breaker Step off21/LConn1
  Delta-Connected Load16/LConn1 -- Circuit Breaker Step off25/RConn1
  Simulink-PS Converter23/RConn1 -- Circuit Breaker Step off23/LConn1
  Delta-Connected Load15/LConn1 -- Circuit Breaker Step off21/RConn1
  Delta-Connected Load14/LConn1 -- Circuit Breaker Step off24/RConn1
  Simulink-PS Converter25/RConn1 -- Circuit Breaker Step off24/LConn1
  Simulink-PS Converter24/RConn1 -- Circuit Breaker Step off22/LConn1
  Delta-Connected Load13/LConn1 -- Circuit Breaker Step off22/RConn1
  Circuit Breaker Step off26/LConn2 -- Circuit Breaker Step off27/LConn2 -- Circuit Breaker Step off29/LConn2 -- Circuit Breaker Step off30/LConn2 -- Circuit Breaker Step off28/RConn1
  Simulink-PS Converter27/RConn1 -- Circuit Breaker Step off30/LConn1
  Delta-Connected Load20/LConn1 -- Circuit Breaker Step off30/RConn1
  Simulink-PS Converter28/RConn1 -- Circuit Breaker Step off28/LConn1
  Circuit Breaker Step off8/LConn2 -- Circuit Breaker Step off33/RConn1 -- Circuit Breaker Step off32/LConn2
  Simulink-PS Converter33/RConn1 -- Circuit Breaker Step off33/LConn1
  Simulink-PS Converter34/RConn1 -- Circuit Breaker Step off32/LConn1
  Delta-Connected Load21/LConn1 -- Circuit Breaker Step off32/RConn1
  Delta-Connected Load17/LConn1 -- Circuit Breaker Step off26/RConn1
  Simulink-PS Converter26/RConn1 -- Circuit Breaker Step off26/LConn1
  Delta-Connected Load18/LConn1 -- Circuit Breaker Step off29/RConn1
  Simulink-PS Converter29/RConn1 -- Circuit Breaker Step off27/LConn1
  Delta-Connected Load19/LConn1 -- Circuit Breaker Step off27/RConn1
  Simulink-PS Converter30/RConn1 -- Circuit Breaker Step off29/LConn1
  Simulink-PS Converter1/RConn1 -- Circuit Breaker Step off3/LConn1
  Delta-Connected Load8/LConn1 -- Circuit Breaker Step off3/RConn1
  Delta-Connected Load22/LConn1 -- Circuit Breaker Step off8/RConn1
  Simulink-PS Converter8/RConn1 -- Circuit Breaker Step off8/LConn1
  Constant load/LConn1 -- Circuit Breaker Step off31/RConn1
  Simulink-PS Converter31/RConn1 -- Circuit Breaker Step off31/LConn1

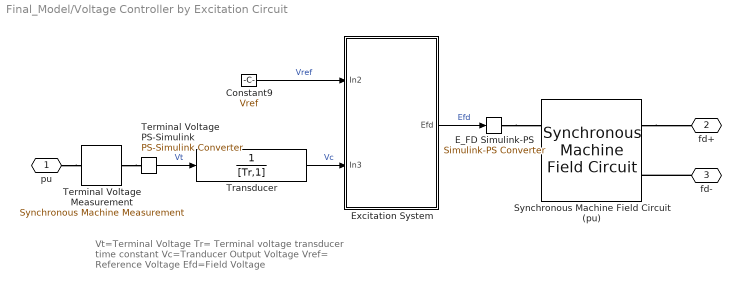
== system Final_Model/Voltage Controller by Excitation Circuit ==
  note: Vt=Terminal Voltage
      | Tr= Terminal voltage transducer time constant
      | Vc=Tranducer Output Voltage
      | Vref= Reference Voltage
      | Efd=Field Voltage
  Constant9 : Constant  Value=Vref
  "E_FD Simulink-PS " : nesl_utility/Simulink-PS Converter  PhysicalDomain=network_engine_domain  SubClassName=ps_input  LeftPortType=input  RightPortType=output  PseudoPeriodic=off  Frequencies=[]  NoiseDistribution=none  NoiseParameters=[]  Unit=1  AffineConversion=off  FilteringAndDerivatives=provide  SimscapeFilterOrder=1  InputFilterTimeConstant=.001  UdotUserProvided=0
      settings: SourceProductBaseCode=MT,SS
  Excitation System : Subsystem
  Synchronous Machine Field Circuit (pu) : ee_lib/Electromechanical/Synchronous/Synchronous Machine Field Circuit  unit_option=ee.enum.unit.pu  SRated=555e6 V*A  FRated=60 Hz  fieldCircuitParameterization_option=2  baseEfd=92.95 V  baseIfd=1300 A  parameterization_option=2  Ladu=1.66  Rfd=0.0006  Xl=0.15  Xd=1.81  Xdd=0.3  Xddd=0.23  d_option=ee.enum.circuit.open  Td0d=8 s  Tdd=1.3260 s  Td0dd=0.03 s  Tddd=0.0230 s
      settings: SourceProductBaseCode=PS  InternalSimscapePortConfiguration="{\"Bottom\":[],\"Left\":[{\"id\":\"Efd_pu\",\"label\":\"Efd_pu\",\"type\":\"input\"},{\"id\":\"Ifd_pu\",\"label\":\"Ifd_pu\",\"type\":\"output\"}],\"Right\":[{\"id\":\"fd_p\",\"label\":\"fd+\",\"type\":\"foundation.electrical.electrical\"},{\"id\":\"fd_n\",\"label\":\"fd-\",\"type\":\"foundation.electrical.electrical\"}],\"Top\":[]}"
  Terminal Voltage Measurement : ee_lib/Electromechanical/Synchronous/Synchronous Machine Measurement  output_idx=14
      settings: SourceProductBaseCode=PS  InternalSimscapePortConfiguration="{\"Bottom\":[],\"Left\":[{\"id\":\"pu_input\",\"label\":\"pu\",\"type\":\"input\"}],\"Right\":[{\"id\":\"pu_output\",\"label\":\"o\",\"type\":\"output\"}],\"Top\":[]}"
  Terminal Voltage PS-Simulink : nesl_utility/PS-Simulink Converter  PhysicalDomain=network_engine_domain  SubClassName=ps_output  LeftPortType=input  RightPortType=output  PseudoPeriodic=off  Frequencies=[]  Unit=1  AffineConversion=off
      settings: SourceProductBaseCode=MT,SS
  Transducer : TransferFcn  Denominator=[Tr,1]
  pu : PMIOPort  Side=Left
  fd+ : PMIOPort  Port=2  Side=Right
  fd- : PMIOPort  Port=3  Side=Right
  wires:
  Excitation System/1(Efd) -> "E_FD Simulink-PS "/1  "Efd"
  Constant9/1 -> Excitation System/1(In2)  "Vref"
  Transducer/1 -> Excitation System/2(In3)  "Vc"
  Terminal Voltage PS-Simulink/1 -> Transducer/1  "Vt"
  connections:
  Terminal Voltage Measurement/RConn1 -- Terminal Voltage PS-Simulink/LConn1
  pu/RConn1 -- Terminal Voltage Measurement/LConn1
  Synchronous Machine Field Circuit (pu)/RConn1 -- fd+/RConn1
  fd-/RConn1 -- Synchronous Machine Field Circuit (pu)/RConn2
  "E_FD Simulink-PS "/RConn1 -- Synchronous Machine Field Circuit (pu)/LConn1

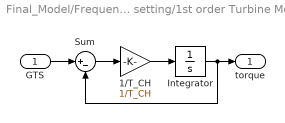
== system Final_Model/Frequency Controller by Governor set point setting/1st order Turbine Model ==
  GTS : Inport
  1/T_CH : Gain  Gain=1/T_CH
  Integrator : Integrator  InitialCondition=pu_torque0
  Sum : Sum  Inputs=|+-
  torque : Outport  VectorParamsAs1DForOutWhenUnconnected=off
  wires:
  GTS/1 -> Sum/1
  Sum/1 -> 1/T_CH/1
  1/T_CH/1 -> Integrator/1
  Integrator/1 -> Sum/2, torque/1

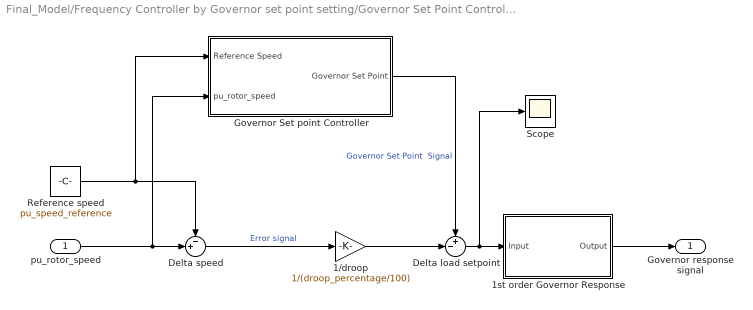
== system Final_Model/Frequency Controller by Governor set point setting/Governor Set Point Controller ==
  pu_rotor_speed : Inport
  1/droop : Gain  Gain=1/(droop_percentage/100)
  1st order Governor Response : Subsystem
  Delta load setpoint : Sum  Inputs=+-|
  Delta speed : Sum  Inputs=-+|
  Governor Set point Controller : Subsystem
  Reference speed : Constant  Value=pu_speed_reference
  Scope : Scope
  Governor response signal : Outport  VectorParamsAs1DForOutWhenUnconnected=off
  wires:
  Reference speed/1 -> Governor Set point Controller/1(Reference Speed), Delta speed/1
  Delta speed/1 -> 1/droop/1  "Error signal"
  pu_rotor_speed/1 -> Governor Set point Controller/2(pu_rotor_speed), Delta speed/2
  1/droop/1 -> Delta load setpoint/2
  Delta load setpoint/1 -> Scope/1, 1st order Governor Response/1(Input)
  1st order Governor Response/1(Output) -> Governor response signal/1
  Governor Set point Controller/1(Governor Set Point) -> Delta load setpoint/1  "Governor Set Point  Signal"
